simulink model "flapping_wing_attitude_plant_v7_framework_refstyle"  (R2025b)
settings: Solver=ode45  StartTime=0.0  StopTime=5  MaxStep=0.001  RelTol=1e-3
settings Model: Creator=Administrator  LastModifiedBy=Administrator

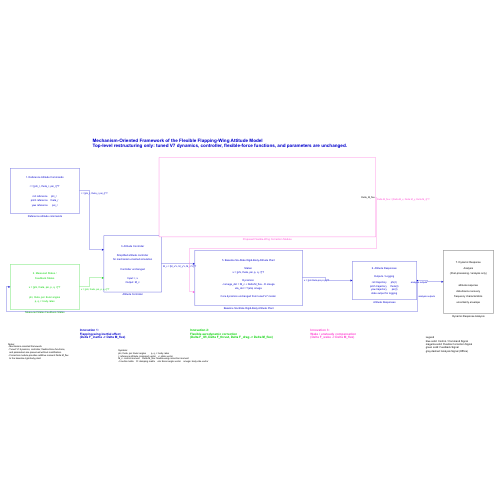
[thumbnail: Simulink's stored preview of the top-level diagram]
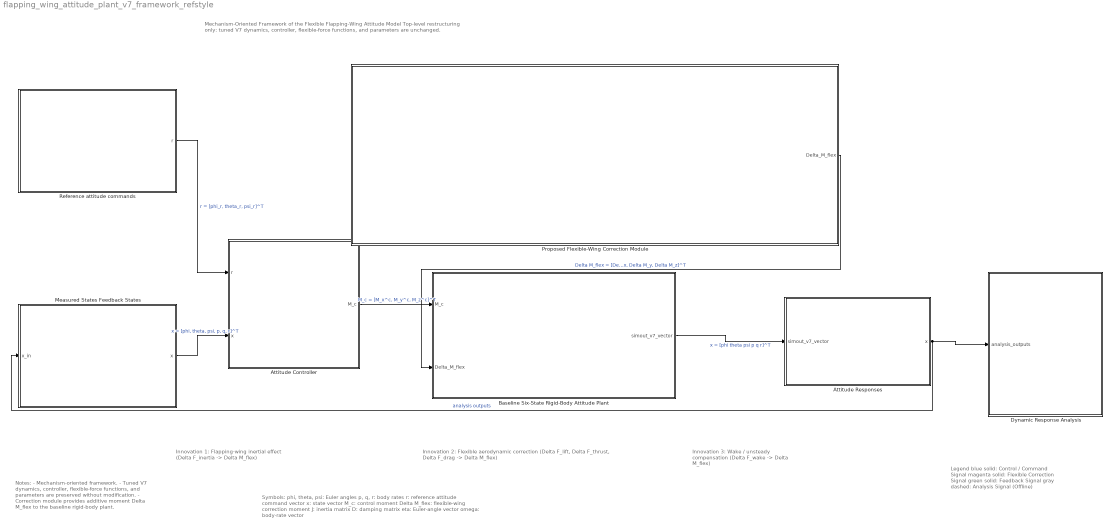
== system flapping_wing_attitude_plant_v7_framework_refstyle ==
  note: Mechanism-Oriented Framework of the Flexible Flapping-Wing Attitude Model
      | Top-level restructuring only: tuned V7 dynamics, controller, flexible-force functions, and parameters are unchanged.
  note: Innovation 1:
      | Flapping-wing inertial effect
      | (Delta F_inertia -> Delta M_flex)
  note: Innovation 2:
      | Flexible aerodynamic correction
      | (Delta F_lift, Delta F_thrust, Delta F_drag -> Delta M_flex)
  note: Innovation 3:
      | Wake / unsteady compensation
      | (Delta F_wake -> Delta M_flex)
  note: Legend
      | blue solid: Control / Command Signal
      | magenta solid: Flexible Correction Signal
      | green solid: Feedback Signal
      | gray dashed: Analysis Signal (Offline)
  note: Notes:
      | - Mechanism-oriented framework.
      | - Tuned V7 dynamics, controller, flexible-force functions,
      |   and parameters are preserved without modification.
      | - Correction module provides additive moment Delta M_flex
      |   to the baseline rigid-body plant.
  note: Symbols:
      | phi, theta, psi: Euler angles        p, q, r: body rates
      | r: reference attitude command vector    x: state vector
      | M_c: control moment    Delta M_flex: flexible-wing correction moment
      | J: inertia matrix    D: damping matrix    eta: Euler-angle vector    omega: body-rate vector
  Attitude Controller : Subsystem
      mask Display: color('blue');text(0.5,0.820,'3. Attitude Controller','horizontalAlignment','center');text(0.5,0.660,'Simplified attitude controller','horizontalAlignment','center');text(0.5,0.580,'for mechanism-oriented simulation','horizontalAlignment','center');text(0.5,0.420,'Controller unchanged','horizontalAlignment','center');text(0.5,0.260,'Input: r, x','horizontalAlignment','center');text(0.5,0.180,'Output: M_c','horizontalAlignment','center');
  Attitude Responses : Subsystem
      mask Display: color('blue');text(0.5,0.820,'6. Attitude Responses','horizontalAlignment','center');text(0.5,0.637,'Outputs / Logging','horizontalAlignment','center');text(0.5,0.454,'roll trajectory      phi(t)','horizontalAlignment','center');text(0.5,0.363,'pitch trajectory     theta(t)','horizontalAlignment','center');text(0.5,0.271,'yaw trajectory       psi(t)','horizontalAlignment','center');text(0.5,0.180,'state output for logging','horizontalAlignment','center');
  Baseline Six-State Rigid-Body Attitude Plant : Subsystem
      mask Display: color('blue');text(0.5,0.820,'5. Baseline Six-State Rigid-Body Attitude Plant','horizontalAlignment','center');text(0.5,0.678,'States:','horizontalAlignment','center');text(0.5,0.607,'x = [phi, theta, psi, p, q, r]^T','horizontalAlignment','center');text(0.5,0.464,'Dynamics:','horizontalAlignment','center');text(0.5,0.393,'J omega_dot = M_c + Delta M_flex - D omega','horizontalAlignment','center');text(0.5,0.322,'eta_dot = T(eta) omega','horizontalAlignment','center');text(0.5,0.180,'Core dynamics unchanged from tuned V7 model.','horizontalAlignment','center');
  Dynamic Response Analysis : Subsystem
      mask Display: color('black');text(0.5,0.820,'7. Dynamic Response','horizontalAlignment','center');text(0.5,0.729,'Analysis','horizontalAlignment','center');text(0.5,0.637,'(Post-processing / analysis only)','horizontalAlignment','center');text(0.5,0.454,'attitude response','horizontalAlignment','center');text(0.5,0.363,'disturbance recovery','horizontalAlignment','center');text(0.5,0.271,'frequency characteristics','horizontalAlignment','center');text(0.5,0.180,'uncertainty envelope','horizontalAlignment','center');
  Measured States Feedback States : Subsystem
      mask Display: color('green');text(0.5,0.820,'2. Measured States /','horizontalAlignment','center');text(0.5,0.713,'Feedback States','horizontalAlignment','center');text(0.5,0.500,'x = [phi, theta, psi, p, q, r]^T','horizontalAlignment','center');text(0.5,0.287,'phi, theta, psi: Euler angles','horizontalAlignment','center');text(0.5,0.180,'p, q, r: body rates','horizontalAlignment','center');
  Proposed Flexible-Wing Correction Module : Subsystem
  Reference attitude commands : Subsystem
      mask Display: color('blue');text(0.5,0.820,'1. Reference Attitude Commands','horizontalAlignment','center');text(0.5,0.607,'r = [phi_r, theta_r, psi_r]^T','horizontalAlignment','center');text(0.5,0.393,'roll reference     phi_r','horizontalAlignment','center');text(0.5,0.287,'pitch reference    theta_r','horizontalAlignment','center');text(0.5,0.180,'yaw reference      psi_r','horizontalAlignment','center');
  wires:
  Reference attitude commands/1(r) -> Attitude Controller/1(r)  "r = [phi_r, theta_r, psi_r]^T"
  Attitude Controller/1(M_c) -> Baseline Six-State Rigid-Body Attitude Plant/1(M_c)  "M_c = [M_x^c, M_y^c, M_z^c]^T"
  Baseline Six-State Rigid-Body Attitude Plant/1(simout_v7_vector) -> Attitude Responses/1(simout_v7_vector)  "x = [phi theta psi p q r]^T"
  Proposed Flexible-Wing Correction Module/1(Delta_M_flex) -> Baseline Six-State Rigid-Body Attitude Plant/2(Delta_M_flex)  "Delta M_flex = [Delta M_x, Delta M_y, Delta M_z]^T"
  Attitude Responses/1(x) -> Measured States Feedback States/1(x_in), Dynamic Response Analysis/1(analysis_outputs)  "analysis outputs"
  Measured States Feedback States/1(x) -> Attitude Controller/2(x)  "x = [phi, theta, psi, p, q, r]^T"

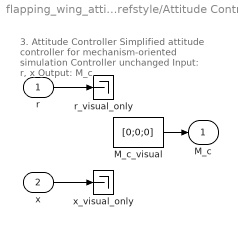
== system flapping_wing_attitude_plant_v7_framework_refstyle/Attitude Controller ==
  note: 3. Attitude Controller
      |
      | Simplified attitude controller
      | for mechanism-oriented simulation
      |
      | Controller unchanged
      |
      | Input: r, x
      | Output: M_c
  r : Inport
  x : Inport  Port=2
  M_c_visual : Constant  Value=[0;0;0]
  r_visual_only : Terminator
  x_visual_only : Terminator
  M_c : Outport
  wires:
  r/1 -> r_visual_only/1
  x/1 -> x_visual_only/1
  M_c_visual/1 -> M_c/1

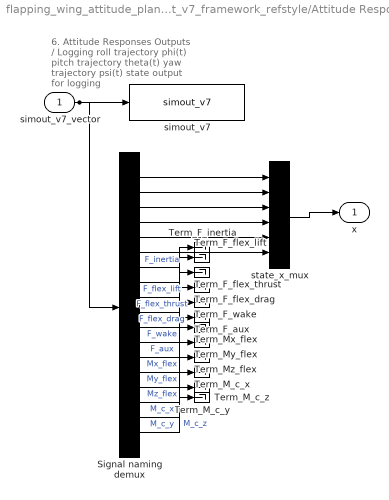
== system flapping_wing_attitude_plant_v7_framework_refstyle/Attitude Responses ==
  note: 6. Attitude Responses
      |
      | Outputs / Logging
      |
      | roll trajectory      phi(t)
      | pitch trajectory     theta(t)
      | yaw trajectory       psi(t)
      | state output for logging
  simout_v7_vector : Inport
  Signal naming demux : Demux  Outputs=18
  Term_F_aux : Terminator
  Term_F_flex_drag : Terminator
  Term_F_flex_lift : Terminator
  Term_F_flex_thrust : Terminator
  Term_F_inertia : Terminator
  Term_F_wake : Terminator
  Term_M_c_x : Terminator
  Term_M_c_y : Terminator
  Term_M_c_z : Terminator
  Term_Mx_flex : Terminator
  Term_My_flex : Terminator
  Term_Mz_flex : Terminator
  simout_v7 : ToWorkspace  VariableName=simout_v7  SaveFormat=Timeseries  SampleTime=-1
  state_x_mux : Mux  Inputs=6
  x : Outport
  wires:
  simout_v7_vector/1 -> simout_v7/1, Signal naming demux/1
  Signal naming demux/1 -> state_x_mux/1
  Signal naming demux/2 -> state_x_mux/2
  Signal naming demux/3 -> state_x_mux/3
  Signal naming demux/4 -> state_x_mux/4
  Signal naming demux/5 -> state_x_mux/5
  Signal naming demux/6 -> state_x_mux/6
  state_x_mux/1 -> x/1
  Signal naming demux/7 -> Term_F_inertia/1  "F_inertia"
  Signal naming demux/8 -> Term_F_flex_lift/1  "F_flex_lift"
  Signal naming demux/9 -> Term_F_flex_thrust/1  "F_flex_thrust"
  Signal naming demux/10 -> Term_F_flex_drag/1  "F_flex_drag"
  Signal naming demux/11 -> Term_F_wake/1  "F_wake"
  Signal naming demux/12 -> Term_F_aux/1  "F_aux"
  Signal naming demux/13 -> Term_Mx_flex/1  "Mx_flex"
  Signal naming demux/14 -> Term_My_flex/1  "My_flex"
  Signal naming demux/15 -> Term_Mz_flex/1  "Mz_flex"
  Signal naming demux/16 -> Term_M_c_x/1  "M_c_x"
  Signal naming demux/17 -> Term_M_c_y/1  "M_c_y"
  Signal naming demux/18 -> Term_M_c_z/1  "M_c_z"

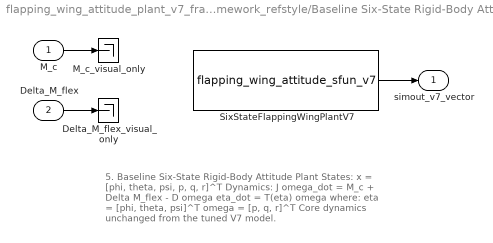
== system flapping_wing_attitude_plant_v7_framework_refstyle/Baseline Six-State Rigid-Body Attitude Plant ==
  note: 5. Baseline Six-State Rigid-Body Attitude Plant
      |
      | States:
      | x = [phi, theta, psi, p, q, r]^T
      |
      | Dynamics:
      | J omega_dot = M_c + Delta M_flex - D omega
      | eta_dot = T(eta) omega
      |
      | where:
      | eta = [phi, theta, psi]^T
      | omega = [p, q, r]^T
      |
      | Core dynamics unchanged from the tuned V7 model.
  M_c : Inport
  Delta_M_flex : Inport  Port=2
  Delta_M_flex_visual_only : Terminator
  M_c_visual_only : Terminator
  SixStateFlappingWingPlantV7 : M-S-Function  FunctionName=flapping_wing_attitude_sfun_v7
  simout_v7_vector : Outport
  wires:
  M_c/1 -> M_c_visual_only/1
  Delta_M_flex/1 -> Delta_M_flex_visual_only/1
  SixStateFlappingWingPlantV7/1 -> simout_v7_vector/1

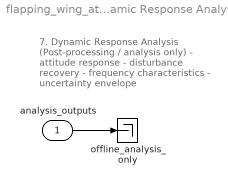
== system flapping_wing_attitude_plant_v7_framework_refstyle/Dynamic Response Analysis ==
  note: 7. Dynamic Response
      | Analysis
      | (Post-processing / analysis only)
      |
      | - attitude response
      | - disturbance recovery
      | - frequency characteristics
      | - uncertainty envelope
  analysis_outputs : Inport
  offline_analysis_only : Terminator
  wires:
  analysis_outputs/1 -> offline_analysis_only/1

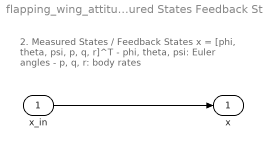
== system flapping_wing_attitude_plant_v7_framework_refstyle/Measured States Feedback States ==
  note: 2. Measured States / Feedback States
      |
      | x = [phi, theta, psi, p, q, r]^T
      |
      | - phi, theta, psi: Euler angles
      | - p, q, r: body rates
  x_in : Inport
  x : Outport
  wires:
  x_in/1 -> x/1

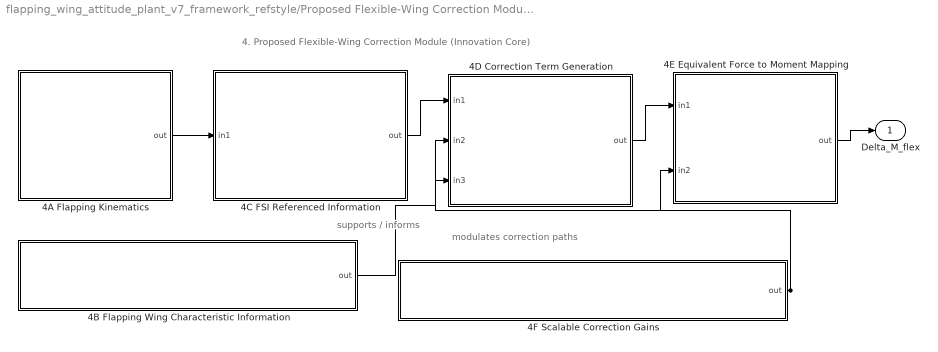
== system flapping_wing_attitude_plant_v7_framework_refstyle/Proposed Flexible-Wing Correction Module ==
  note: 4. Proposed Flexible-Wing Correction Module (Innovation Core)
  note: supports / informs
  note: modulates correction paths
  4A Flapping Kinematics : Subsystem
      mask Display: color('magenta');text(0.5,0.820,'4A. Flapping','horizontalAlignment','center');text(0.5,0.713,'Kinematics','horizontalAlignment','center');text(0.5,0.500,'phi_w(t)','horizontalAlignment','center');text(0.5,0.393,'phi_dot_w(t)','horizontalAlignment','center');text(0.5,0.287,'phi_ddot_w(t)','horizontalAlignment','center');text(0.5,0.180,'A0, f_flap','horizontalAlignment','center');
  4B Flapping Wing Characteristic Information : Subsystem
      mask Display: color('magenta');text(0.5,0.820,'4B. Flapping-Wing','horizontalAlignment','center');text(0.5,0.607,'Characteristic Information','horizontalAlignment','center');text(0.5,0.180,'b, c, S, AR, wing mass/inertia, k, Re','horizontalAlignment','center');
  4C FSI Referenced Information : Subsystem
      mask Display: color('magenta');text(0.5,0.820,'4C. FSI-Referenced','horizontalAlignment','center');text(0.5,0.692,'Aerodynamic / Structural Information','horizontalAlignment','center');text(0.5,0.436,'flexible deformation','horizontalAlignment','center');text(0.5,0.308,'aerodynamic trend extraction','horizontalAlignment','center');text(0.5,0.180,'force correction identification','horizontalAlignment','center');
  4D Correction Term Generation : Subsystem
      mask Display: color('magenta');text(0.5,0.820,'4D. Correction Term','horizontalAlignment','center');text(0.5,0.729,'Generation','horizontalAlignment','center');text(0.5,0.546,'Delta F_inertia','horizontalAlignment','center');text(0.5,0.454,'Delta F_lift','horizontalAlignment','center');text(0.5,0.363,'Delta F_thrust','horizontalAlignment','center');text(0.5,0.271,'Delta F_drag','horizontalAlignment','center');text(0.5,0.180,'Delta F_wake','horizontalAlignment','center');
  4E Equivalent Force to Moment Mapping : Subsystem
      mask Display: color('magenta');text(0.5,0.820,'4E. Equivalent','horizontalAlignment','center');text(0.5,0.692,'Force-to-Moment Mapping','horizontalAlignment','center');text(0.5,0.436,'Delta M_x','horizontalAlignment','center');text(0.5,0.308,'Delta M_y','horizontalAlignment','center');text(0.5,0.180,'Delta M_z','horizontalAlignment','center');
  4F Scalable Correction Gains : Subsystem
      mask Display: color('magenta');text(0.5,0.820,'4F. Scalable Correction Gains','horizontalAlignment','center');text(0.5,0.180,'s_inertia, s_flex, s_wake','horizontalAlignment','center');
  Delta_M_flex : Outport
  wires:
  4A Flapping Kinematics/1(out) -> 4C FSI Referenced Information/1(in1)
  4C FSI Referenced Information/1(out) -> 4D Correction Term Generation/1(in1)
  4B Flapping Wing Characteristic Information/1(out) -> 4D Correction Term Generation/2(in2)
  4F Scalable Correction Gains/1(out) -> 4D Correction Term Generation/3(in3), 4E Equivalent Force to Moment Mapping/2(in2)
  4D Correction Term Generation/1(out) -> 4E Equivalent Force to Moment Mapping/1(in1)
  4E Equivalent Force to Moment Mapping/1(out) -> Delta_M_flex/1

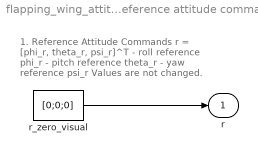
== system flapping_wing_attitude_plant_v7_framework_refstyle/Reference attitude commands ==
  note: 1. Reference Attitude Commands
      |
      | r = [phi_r, theta_r, psi_r]^T
      |
      | - roll reference     phi_r
      | - pitch reference    theta_r
      | - yaw reference      psi_r
      |
      | Values are not changed.
  r_zero_visual : Constant  Value=[0;0;0]
  r : Outport
  wires:
  r_zero_visual/1 -> r/1

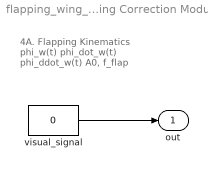
== system flapping_wing_attitude_plant_v7_framework_refstyle/Proposed Flexible-Wing Correction Module/4A Flapping Kinematics ==
  note: 4A. Flapping
      | Kinematics
      |
      | phi_w(t)
      | phi_dot_w(t)
      | phi_ddot_w(t)
      | A0, f_flap
  visual_signal : Constant  Value=0
  out : Outport
  wires:
  visual_signal/1 -> out/1

== system flapping_wing_attitude_plant_v7_framework_refstyle/Proposed Flexible-Wing Correction Module/4B Flapping Wing Characteristic Information ==
  note: 4B. Flapping-Wing
      | Characteristic Information
      |
      | b, c, S, AR, wing mass/inertia, k, Re
  visual_signal : Constant  Value=0
  out : Outport
  wires:
  visual_signal/1 -> out/1

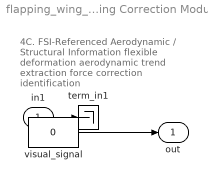
== system flapping_wing_attitude_plant_v7_framework_refstyle/Proposed Flexible-Wing Correction Module/4C FSI Referenced Information ==
  note: 4C. FSI-Referenced
      | Aerodynamic / Structural Information
      |
      | flexible deformation
      | aerodynamic trend extraction
      | force correction identification
  in1 : Inport
  term_in1 : Terminator
  visual_signal : Constant  Value=0
  out : Outport
  wires:
  in1/1 -> term_in1/1
  visual_signal/1 -> out/1

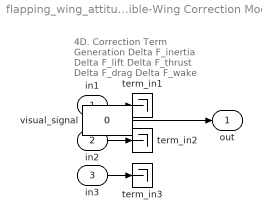
== system flapping_wing_attitude_plant_v7_framework_refstyle/Proposed Flexible-Wing Correction Module/4D Correction Term Generation ==
  note: 4D. Correction Term
      | Generation
      |
      | Delta F_inertia
      | Delta F_lift
      | Delta F_thrust
      | Delta F_drag
      | Delta F_wake
  in1 : Inport
  in2 : Inport  Port=2
  in3 : Inport  Port=3
  term_in1 : Terminator
  term_in2 : Terminator
  term_in3 : Terminator
  visual_signal : Constant  Value=0
  out : Outport
  wires:
  in1/1 -> term_in1/1
  in2/1 -> term_in2/1
  in3/1 -> term_in3/1
  visual_signal/1 -> out/1

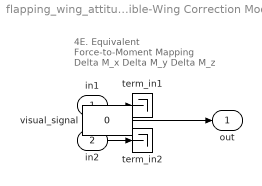
== system flapping_wing_attitude_plant_v7_framework_refstyle/Proposed Flexible-Wing Correction Module/4E Equivalent Force to Moment Mapping ==
  note: 4E. Equivalent
      | Force-to-Moment Mapping
      |
      | Delta M_x
      | Delta M_y
      | Delta M_z
  in1 : Inport
  in2 : Inport  Port=2
  term_in1 : Terminator
  term_in2 : Terminator
  visual_signal : Constant  Value=0
  out : Outport
  wires:
  in1/1 -> term_in1/1
  in2/1 -> term_in2/1
  visual_signal/1 -> out/1

== system flapping_wing_attitude_plant_v7_framework_refstyle/Proposed Flexible-Wing Correction Module/4F Scalable Correction Gains ==
  note: 4F. Scalable Correction Gains
      |
      | s_inertia, s_flex, s_wake
  visual_signal : Constant  Value=0
  out : Outport
  wires:
  visual_signal/1 -> out/1
